simulink model "tpi2parallel"  (R2017b)
settings: Solver=ode8  StartTime=0.0  StopTime=0.1  FixedStep=1e-6  MaxStep=1e-4  RelTol=1e-3
values from neighbouring files (symbols this model uses):
  dcin = 547.66    [tpi2parallelrunner.m]    (also in tpi2seriesrunner.m = 20; tpireloadedrunner.m)
  fdclinkcap = 100e-6    (= 0.0001)    [tpi2parallelrunner.m]    (also in tpi2seriesrunner.m = 0.01; tpireloadedrunner.m = 0.01)
  fdclinkres = 1e-6    (= 1e-06)    [tpi2parallelrunner.m]    (also in tpi2seriesrunner.m; tpireloadedrunner.m)
  FLload = FXload/freffreq    [tpi2parallelrunner.m]    (also in tpi2seriesrunner.m = 0.002; tpireloadedrunner.m)
  fma = 0.9    [tpi2parallelrunner.m]    (also in tpi2seriesrunner.m; tpireloadedrunner.m)
  freffreq = 2*pi*50    (= 314.159265359)    [tpi2parallelrunner.m]    (also in tpi2seriesrunner.m; tpireloadedrunner.m)
  FRload = FZload*Load_Power_Factor    [tpi2parallelrunner.m]    (also in tpi2seriesrunner.m = 5; tpireloadedrunner.m = n*FZload*Load_Power_Factor)
  Rin = 1    [tpi2parallelrunner.m]    (also in tpi2seriesrunner.m = 1e-16; tpireloadedrunner.m)
  SLload = SXload/sreffreq    [tpi2parallelrunner.m]    (also in tpi2seriesrunner.m = 0.002; tpireloadedrunner.m)
  sma = 0.9    [tpi2parallelrunner.m]    (also in tpi2seriesrunner.m; tpireloadedrunner.m)
  sreffreq = 2*pi*50    (= 314.159265359)    [tpi2parallelrunner.m]    (also in tpi2seriesrunner.m; tpireloadedrunner.m)
  SRload = SZload*Load_Power_Factor    [tpi2parallelrunner.m]    (also in tpi2seriesrunner.m = 5; tpireloadedrunner.m = n*SZload*Load_Power_Factor)
undefined symbols (not defined in the file or in its folder): fdclink1cap
libraries: powerlib x39, simulink x6, dspstat3 x6, powerlib_meascontrol x5
settings Model: Creator=Orhun  LastModifiedBy=Orhun
settings SolverCC: ZeroCrossAlgorithm=Adaptive
settings DebuggingCC: MaxConsecutiveZCsMsg=none

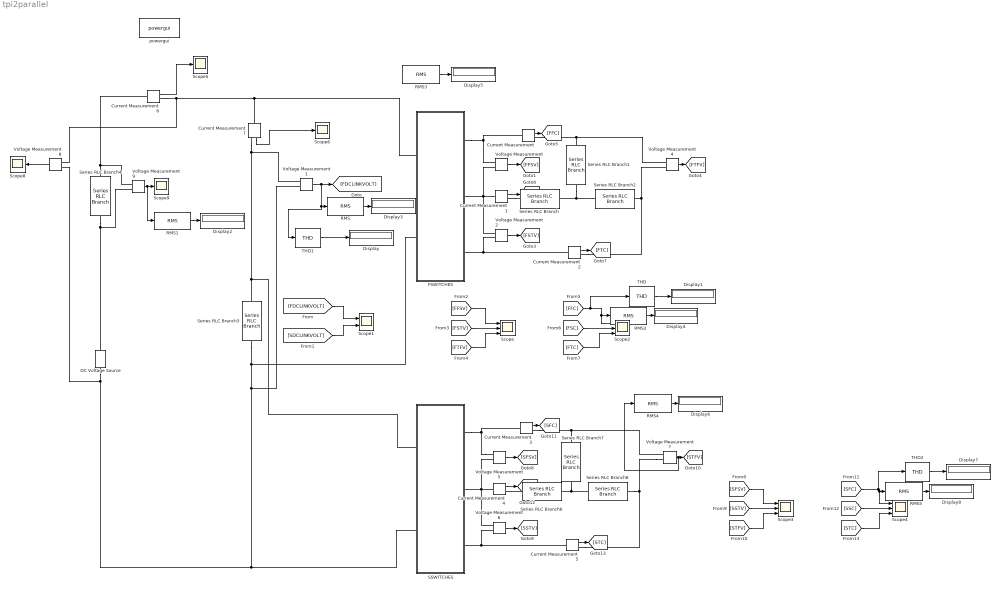
== system tpi2parallel ==
  Current Measurement{,1..7} (8 alike) : powerlib/Measurements/Current Measurement  PhasorSimulation=off  OutputType=Complex  PSBequivalent=0
  DC Voltage Source : powerlib/Electrical Sources/DC Voltage Source  Amplitude=dcin  Measurements=None
  Display{,1..8} (9 alike) : Display
  FSWITCHES : Subsystem
  RMS : dspstat3/RMS  run=on  directionMode=Each column  dimension=1  InputProcessing=Columns as channels (frame based)  reset_popup=None
  RMS1 : dspstat3/RMS  run=off  directionMode=Each column  dimension=1  InputProcessing=Columns as channels (frame based)  reset_popup=None
  RMS2 : dspstat3/RMS  run=on  directionMode=Entire input  dimension=1  InputProcessing=Columns as channels (frame based)  reset_popup=None
  RMS3 : dspstat3/RMS  run=off  directionMode=Each column  dimension=1  InputProcessing=Columns as channels (frame based)  reset_popup=None
  RMS4 : dspstat3/RMS  run=on  directionMode=Entire input  dimension=1  InputProcessing=Columns as channels (frame based)  reset_popup=None
  RMS5 : dspstat3/RMS  run=on  directionMode=Entire input  dimension=1  InputProcessing=Columns as channels (frame based)  reset_popup=None
  SSWITCHES : Subsystem
  Scope{,2..4} (4 alike) : Scope  NumInputPorts=3
  Scope1 : Scope  NumInputPorts=2
  Scope{5..6,8..9} (4 alike) : Scope
  Series RLC Branch : powerlib/Elements/Series RLC Branch  LConnTagsString=__new0  RConnTagsString=__new0  BranchType=RL  Resistance=FRload  Inductance=FLload  SetiL0=off  InitialCurrent=0  Capacitance=0  Setx0=off  InitialVoltage=0  Measurements=None
  Series RLC Branch1 : powerlib/Elements/Series RLC Branch  LConnTagsString=__new0  RConnTagsString=__new0  BranchType=RL  Resistance=FRload  Inductance=FLload  SetiL0=off  InitialCurrent=0  Capacitance=0  Setx0=off  InitialVoltage=0  Measurements=None
  Series RLC Branch2 : powerlib/Elements/Series RLC Branch  LConnTagsString=__new0  RConnTagsString=__new0  BranchType=RL  Resistance=FRload  Inductance=FLload  SetiL0=off  InitialCurrent=0  Capacitance=0  Setx0=off  InitialVoltage=0  Measurements=None
  Series RLC Branch3 : powerlib/Elements/Series RLC Branch  LConnTagsString=__new0  RConnTagsString=__new0  BranchType=C  Resistance=fdclinkres  Inductance=0  SetiL0=off  InitialCurrent=0  Capacitance=fdclinkcap  Setx0=off  InitialVoltage=dcin/2  Measurements=None
  Series RLC Branch4 : powerlib/Elements/Series RLC Branch  LConnTagsString=__new0  RConnTagsString=__new0  BranchType=R  Resistance=Rin  Inductance=0  SetiL0=off  InitialCurrent=0  Capacitance=fdclink1cap  Setx0=off  InitialVoltage=0  Measurements=None
  Series RLC Branch6 : powerlib/Elements/Series RLC Branch  LConnTagsString=__new0  RConnTagsString=__new0  BranchType=RL  Resistance=SRload  Inductance=SLload  SetiL0=off  InitialCurrent=0  Capacitance=0  Setx0=off  InitialVoltage=0  Measurements=None
  Series RLC Branch7 : powerlib/Elements/Series RLC Branch  LConnTagsString=__new0  RConnTagsString=__new0  BranchType=RL  Resistance=SRload  Inductance=SLload  SetiL0=off  InitialCurrent=0  Capacitance=0  Setx0=off  InitialVoltage=0  Measurements=None
  Series RLC Branch8 : powerlib/Elements/Series RLC Branch  LConnTagsString=__new0  RConnTagsString=__new0  BranchType=RL  Resistance=SRload  Inductance=SLload  SetiL0=off  InitialCurrent=0  Capacitance=0  Setx0=off  InitialVoltage=0  Measurements=None
  THD : powerlib_meascontrol/Measurements/THD  Freq=50  Ts=0
  THD1 : powerlib_meascontrol/Measurements/THD  Freq=50  Ts=0
  THD2 : powerlib_meascontrol/Measurements/THD  Freq=50  Ts=0
  Voltage Measurement{,1..2,4..9} (9 alike) : powerlib/Measurements/Voltage Measurement  PhasorSimulation=off  OutputType=Complex  PSBequivalent=0
  powergui : powerlib/powergui  Priority=1  SimulationMode=Discrete  SampleTime=1e-6  frequency=60  Iterations=50  frequencyindice=0  Pbase=100e6  ErrMax=1e-4  UnitsV=kV  UnitsW=MW  buscounter=0  FunctionMessages=on  echomessages=off  EnableUseOfTLC=off  CurrentSourceSwitches=off  DisableSnubberDevices=off  DisableRonSwitches=off  DisableVfSwitches=off  DisplayEquations=off  SolverType=Tustin/Backward Euler (TBE)  Interpol=off  ExternalGateDelay=off  methode=off  Ts=100  x0status=blocks  SPID=off  SwTol=0  HookPort=off  RestoreLinks=warning  ResistiveCurrentMeasurement=off  Frange=[0:2:500]  Ylog=off  Xlog=on  ShowGrid=off  save=off  variable=ZData  structure=0  ZoomFFT=off  StartTime=0.0  cycles=1  DisplayStyle=1  fundamental=60  FreqAxis=off  MaxFrequency=1000  frequencyindicesteady=1  RmsSteady=1  display=off
  wires:
  Voltage Measurement1/1 -> RMS/1, THD1/1, [FDCLINKVOLT]
  [FDCLINKVOLT] -> Scope1/1
  [SDCLINKVOLT] -> Scope1/2
  Voltage Measurement/1 -> [FFSV]
  Voltage Measurement2/1 -> [FSTV]
  Voltage Measurement4/1 -> [FTFV]
  Current Measurement/1 -> [FFC]
  Current Measurement1/1 -> [FSC]
  Current Measurement2/1 -> [FTC]
  [FFSV] -> Scope/1
  [FSTV] -> Scope/2
  [FTFV] -> Scope/3
  [FFC] -> THD/1, RMS2/1, Scope2/1
  [SSTV] -> Scope3/2
  [STC] -> Scope4/3
  [STFV] -> Scope3/3
  [SSC] -> Scope4/2
  [SFSV] -> Scope3/1
  [SFC] -> THD2/1, RMS5/1, Scope4/1
  Current Measurement3/1 -> [SFC]
  Current Measurement4/1 -> [SSC]
  Voltage Measurement5/1 -> [SFSV]
  Voltage Measurement6/1 -> [SSTV]
  Current Measurement5/1 -> [STC]
  Voltage Measurement7/1 -> RMS4/1, [STFV]
  Current Measurement6/1 -> Scope5/1
  THD1/1 -> Display/1
  Current Measurement7/1 -> Scope6/1
  THD/1 -> Display1/1
  Voltage Measurement8/1 -> Scope8/1
  Voltage Measurement9/1 -> RMS1/1, Scope9/1
  RMS1/1 -> Display2/1
  RMS/1 -> Display3/1
  RMS2/1 -> Display4/1
  RMS3/1 -> Display5/1
  RMS4/1 -> Display6/1
  [FSC] -> Scope2/2
  [FTC] -> Scope2/3
  THD2/1 -> Display7/1
  RMS5/1 -> Display8/1
  connections:
  Current Measurement6/RConn1 -- Current Measurement7/LConn1 -- FSWITCHES/LConn1 -- Voltage Measurement8/LConn1
  Series RLC Branch4/RConn1 -- Voltage Measurement9/LConn2 -- DC Voltage Source/RConn1
  Voltage Measurement8/LConn2 -- Voltage Measurement1/LConn2 -- FSWITCHES/LConn2 -- Series RLC Branch3/RConn1 -- SSWITCHES/LConn2 -- DC Voltage Source/LConn1
  FSWITCHES/RConn1 -- Current Measurement/LConn1 -- Voltage Measurement/LConn1
  FSWITCHES/RConn2 -- Current Measurement1/LConn1 -- Voltage Measurement2/LConn1 -- Voltage Measurement/LConn2
  Series RLC Branch2/LConn1 -- Current Measurement2/RConn1 -- Voltage Measurement4/LConn1
  Series RLC Branch8/RConn1 -- Series RLC Branch7/LConn1 -- Series RLC Branch6/LConn1
  Current Measurement/RConn1 -- Series RLC Branch1/RConn1 -- Voltage Measurement4/LConn2
  Current Measurement1/RConn1 -- Series RLC Branch/RConn1
  Voltage Measurement2/LConn2 -- Current Measurement2/LConn1 -- FSWITCHES/RConn3
  Current Measurement3/RConn1 -- Series RLC Branch7/RConn1 -- Voltage Measurement7/LConn2
  Voltage Measurement5/LConn1 -- SSWITCHES/RConn1 -- Current Measurement3/LConn1
  Voltage Measurement5/LConn2 -- SSWITCHES/RConn2 -- Current Measurement4/LConn1 -- Voltage Measurement6/LConn1
  Voltage Measurement7/LConn1 -- Series RLC Branch8/LConn1 -- Current Measurement5/RConn1
  Voltage Measurement6/LConn2 -- Current Measurement5/LConn1 -- SSWITCHES/RConn3
  Series RLC Branch6/RConn1 -- Current Measurement4/RConn1
  Current Measurement6/LConn1 -- Voltage Measurement9/LConn1 -- Series RLC Branch4/LConn1
  Voltage Measurement1/LConn1 -- Current Measurement7/RConn1 -- SSWITCHES/LConn1 -- Series RLC Branch3/LConn1
  Series RLC Branch2/RConn1 -- Series RLC Branch1/LConn1 -- Series RLC Branch/LConn1

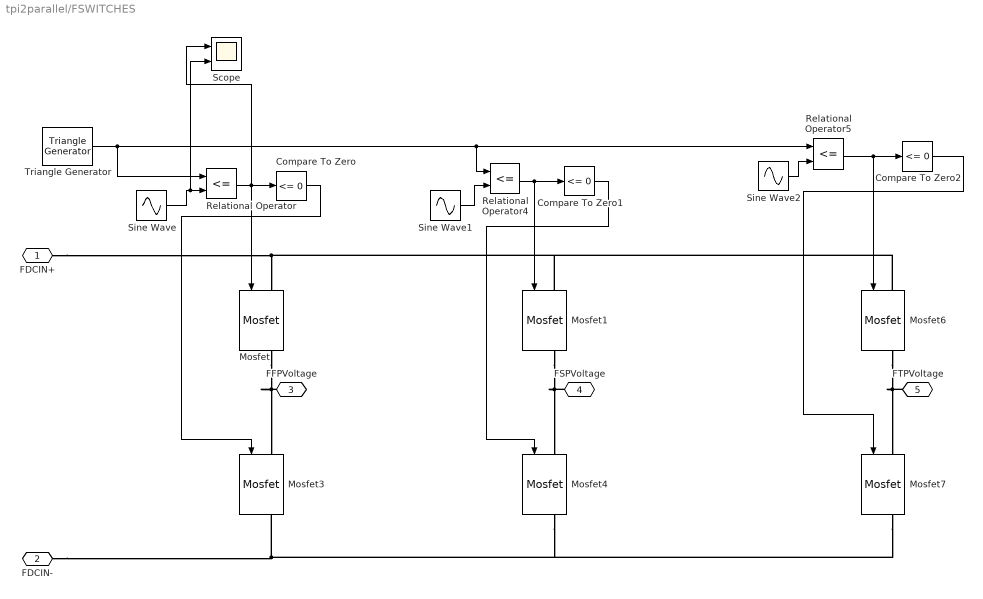
== system tpi2parallel/FSWITCHES ==
  Compare To Zero : simulink/Logic and Bit Operations/Compare To Zero  relop=<=  OutDataTypeStr=boolean
  Compare To Zero1 : simulink/Logic and Bit Operations/Compare To Zero  relop=<=  OutDataTypeStr=boolean
  Compare To Zero2 : simulink/Logic and Bit Operations/Compare To Zero  relop=<=  OutDataTypeStr=boolean
  Mosfet{,1,3..4,6..7} (6 alike) : powerlib/Power Electronics/Mosfet  Ron=2e-3  Lon=0  Rd=0.01  Vfd=0  IC=0  Rs=1e5  Cs=inf  Measurements=on
  Relational Operator : RelationalOperator  Operator=<=  OutDataTypeStr=boolean  RndMeth=Simplest
  Relational Operator4 : RelationalOperator  Operator=<=  OutDataTypeStr=boolean  RndMeth=Simplest
  Relational Operator5 : RelationalOperator  Operator=<=  OutDataTypeStr=boolean  RndMeth=Simplest
  Scope : Scope  NumInputPorts=2
  Sine Wave : Sin  Amplitude=fma  Frequency=freffreq  SampleTime=0
  Sine Wave1 : Sin  Amplitude=fma  Frequency=freffreq  Phase=2*pi/3  SampleTime=0
  Sine Wave2 : Sin  Amplitude=fma  Frequency=freffreq  Phase=4*pi/3  SampleTime=0
  Triangle Generator : powerlib_meascontrol/Pulse & Signal Generators/Triangle Generator  Freq=fswfreq  Phase=90  Ts=1e-6
  FDCIN+ : PMIOPort  Port=1  Side=Left
  FDCIN- : PMIOPort  Port=2  Side=Left
  FFPVoltage : PMIOPort  Port=3  Side=Right
  FSPVoltage : PMIOPort  Port=4  Side=Right
  FTPVoltage : PMIOPort  Port=5  Side=Right
  wires:
  Sine Wave/1 -> Scope/2, Relational Operator/2
  Triangle Generator/1 -> Relational Operator5/1, Relational Operator4/1, Relational Operator/1
  Relational Operator4/1 -> Mosfet1/1, Compare To Zero1/1
  Sine Wave2/1 -> Relational Operator5/2
  Sine Wave1/1 -> Relational Operator4/2
  Relational Operator/1 -> Mosfet/1, Scope/1, Compare To Zero/1
  Compare To Zero/1 -> Mosfet3/1
  Compare To Zero1/1 -> Mosfet4/1
  Compare To Zero2/1 -> Mosfet7/1
  Relational Operator5/1 -> Mosfet6/1, Compare To Zero2/1
  connections:
  Mosfet6/RConn1 -- FTPVoltage/RConn1 -- Mosfet7/LConn1
  Mosfet/RConn1 -- FFPVoltage/RConn1 -- Mosfet3/LConn1
  Mosfet1/RConn1 -- FSPVoltage/RConn1 -- Mosfet4/LConn1
  FDCIN+/RConn1 -- Mosfet6/LConn1 -- Mosfet1/LConn1 -- Mosfet/LConn1
  FDCIN-/RConn1 -- Mosfet4/RConn1 -- Mosfet7/RConn1 -- Mosfet3/RConn1

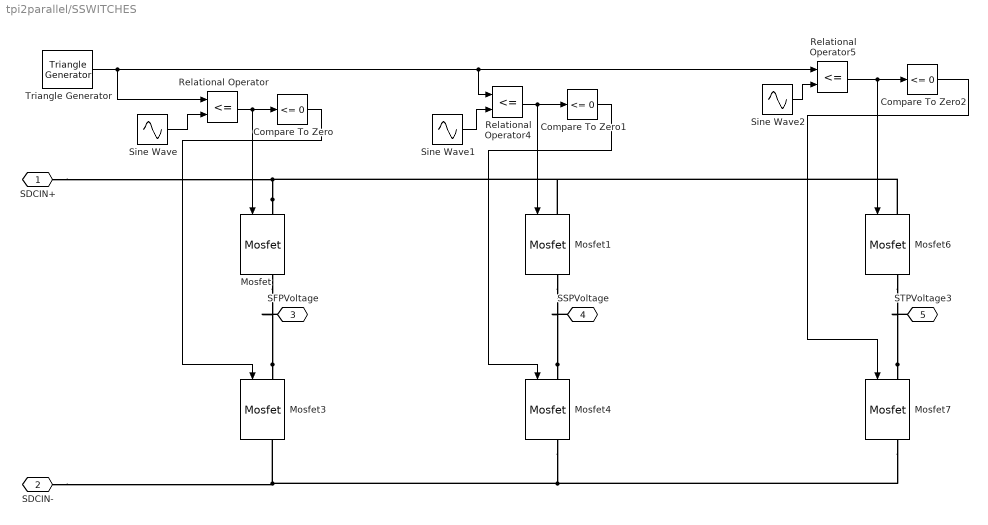
== system tpi2parallel/SSWITCHES ==
  Compare To Zero : simulink/Logic and Bit Operations/Compare To Zero  relop=<=  OutDataTypeStr=boolean
  Compare To Zero1 : simulink/Logic and Bit Operations/Compare To Zero  relop=<=  OutDataTypeStr=boolean
  Compare To Zero2 : simulink/Logic and Bit Operations/Compare To Zero  relop=<=  OutDataTypeStr=boolean
  Mosfet{,1,3..4,6..7} (6 alike) : powerlib/Power Electronics/Mosfet  Ron=2e-3  Lon=0  Rd=0.01  Vfd=0  IC=0  Rs=1e5  Cs=inf  Measurements=on
  Relational Operator : RelationalOperator  Operator=<=  OutDataTypeStr=boolean  RndMeth=Simplest
  Relational Operator4 : RelationalOperator  Operator=<=  OutDataTypeStr=boolean  RndMeth=Simplest
  Relational Operator5 : RelationalOperator  Operator=<=  OutDataTypeStr=boolean  RndMeth=Simplest
  Sine Wave : Sin  Amplitude=sma  Frequency=sreffreq  SampleTime=0
  Sine Wave1 : Sin  Amplitude=sma  Frequency=sreffreq  Phase=2*pi/3  SampleTime=0
  Sine Wave2 : Sin  Amplitude=fma  Frequency=sreffreq  Phase=4*pi/3  SampleTime=0
  Triangle Generator : powerlib_meascontrol/Pulse & Signal Generators/Triangle Generator  Freq=sswfreq  Phase=270  Ts=1e-6
  SDCIN+ : PMIOPort  Port=1  Side=Left
  SDCIN- : PMIOPort  Port=2  Side=Left
  SFPVoltage : PMIOPort  Port=3  Side=Right
  SSPVoltage : PMIOPort  Port=4  Side=Right
  STPVoltage3 : PMIOPort  Port=5  Side=Right
  wires:
  Sine Wave/1 -> Relational Operator/2
  Triangle Generator/1 -> Relational Operator5/1, Relational Operator4/1, Relational Operator/1
  Relational Operator4/1 -> Mosfet1/1, Compare To Zero1/1
  Sine Wave2/1 -> Relational Operator5/2
  Sine Wave1/1 -> Relational Operator4/2
  Relational Operator/1 -> Compare To Zero/1, Mosfet/1
  Compare To Zero/1 -> Mosfet3/1
  Compare To Zero1/1 -> Mosfet4/1
  Compare To Zero2/1 -> Mosfet7/1
  Relational Operator5/1 -> Mosfet6/1, Compare To Zero2/1
  connections:
  Mosfet7/LConn1 -- Mosfet6/RConn1 -- STPVoltage3/RConn1
  Mosfet3/LConn1 -- Mosfet/RConn1 -- SFPVoltage/RConn1
  Mosfet4/LConn1 -- Mosfet1/RConn1 -- SSPVoltage/RConn1
  Mosfet/LConn1 -- SDCIN+/RConn1 -- Mosfet6/LConn1 -- Mosfet1/LConn1
  Mosfet4/RConn1 -- Mosfet3/RConn1 -- SDCIN-/RConn1 -- Mosfet7/RConn1
